simulink library "csu_afm_aerodynamics_lib"  (R2014b)
settings: Solver=ode45  StartTime=0.0  StopTime=10.0  RelTol=1e-3
values from neighbouring files (symbols this model uses):
  AeroData =     [AeroData.mat]
  afm_cg_enable = 1    [csu_afm_aerodynamics_init.m]    (also in unit_test_aero.m = 0)
  afm_forces_enable = 1    [csu_afm_aerodynamics_init.m]
  afm_gust_direction = 0.0    (= 0)    [csu_afm_aerodynamics_init.m]
  afm_gust_length = 1.0    (= 1)    [csu_afm_aerodynamics_init.m]
  afm_gust_magnitude = 0.0    (= 0)    [csu_afm_aerodynamics_init.m]
  afm_gust_number = 1    [csu_afm_aerodynamics_init.m]
  afm_gust_start = 0.0    (= 0)    [csu_afm_aerodynamics_init.m]
  afm_moments_enable = 1    [csu_afm_aerodynamics_init.m]
  afm_winds_enable = 1    [csu_afm_aerodynamics_init.m]    (also in unit_test_aero.m = 0; unit_test_winds.m)
undefined symbols (not defined in the file or in its folder): CM
libraries: simulink_need_slupdate x49, util_common_lib x17, simulink_extras x10, simulink x7, util_quat_lib x6, util_info_lib x2, util_frame_rotation_lib x2
(part 1 of 2)
settings Model: Creator=Mark Agbayani  LastModifiedBy=Mark Wells

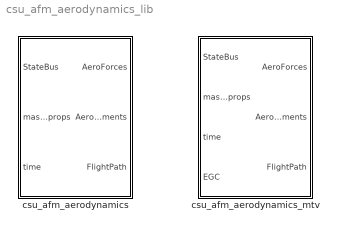
== system csu_afm_aerodynamics_lib ==
  csu_afm_aerodynamics : Subsystem
  csu_afm_aerodynamics_mtv : Subsystem

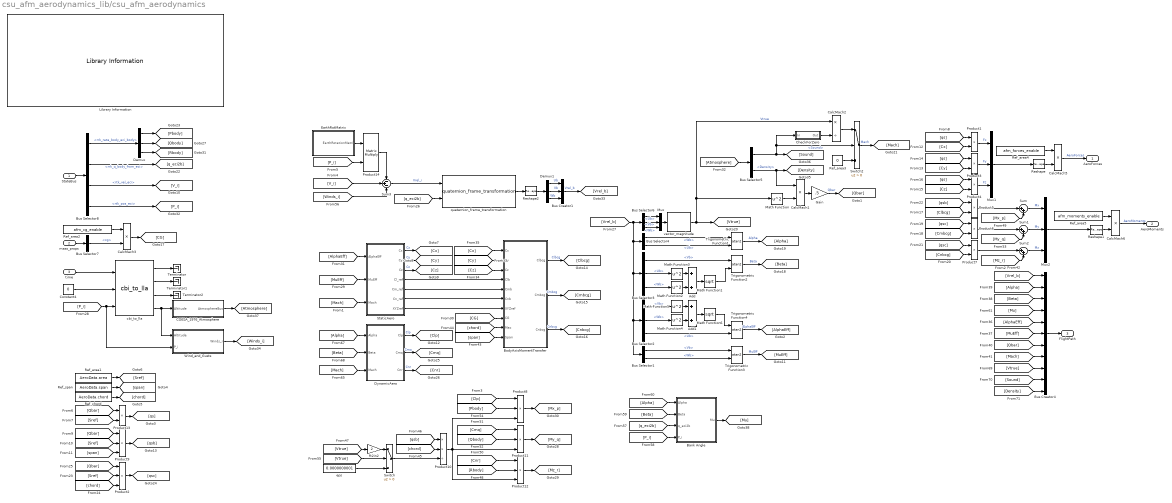
== system csu_afm_aerodynamics_lib/csu_afm_aerodynamics ==
  StateBus : Inport
  mass_props : Inport  Port=2
  time : Inport  Port=3
  Add : Sum
  Add1 : Sum
  Bank Angle : Subsystem
  BodyAxisMomentTransfer : Subsystem
  Bus Creator1 : BusCreator  Inputs=3
  Bus Creator4 : BusCreator  Inputs=11
  Bus Selector1 : BusSelector  OutputSignals=Vb,Wb
  Bus Selector2 : BusSelector  OutputSignals=Vb,Wb,Ub
  Bus Selector3 : BusSelector  OutputSignals=Vb,Ub,Wb
  Bus Selector4 : BusSelector  OutputSignals=Wb,Ub
  Bus Selector5 : BusSelector  OutputSignals=Sound,Density
  Bus Selector6 : BusSelector  OutputSignals=Ub,Vb,Wb
  Bus Selector7 : BusSelector  OutputSignals=cg
  Bus Selector8 : BusSelector  OutputSignals=rrk_rate_body_eci_body,rrk_q_body_from_eci,rtk_vel_eci,rtk_pos_eci
  COESA_1976_Atmosphere : Subsystem  mask(COESA 1976 U.S. Standard Atmosphere){}
      mask help:
      | Committee on Extension to the Standard Atmosphere (COESA) U.S. 1976 Atmosphere Model
      |
      | Computes the atmospheric values of a given geometric  altitude based on the 1976
      | U.S. Standard Atmosphere Model.  This model is valid between -5 km and 1000 km
      | (-16,404 ft and 3,280,840 ft).  Use of this block requires the associated .mat file
      | 'COESA_1976.mat'.
      |
      | Inputs:
      |        Altitude	  [m]   Geometric Altitude
      |
      | Outputs:   AtmosphereBus
      |
      |        SIGNAL NAME          UNITS       DESCRIPTION
      |        GeometricAlt         [m]         Geometric Altitude
      |        GeopotentialAlt      [m]         Geopotential Altitude
      |        Temp_Kinetic         [deg K]     Kinetic Temperature
      |        Temp_Molecular       [deg K]     Molecular Temperature
      |        Pressure             [Pa]        Atmospheric Pressure
      |        PPo                  [unitless]  Pressure / Pressure0
      |        Density              [kg/m^3]    Atmospheric Density
      |        RhoRho0              [unitless]  Rho / Rho0
      |        Sound                [m/s]       Speed of sound, Cs
      |        DynamicViscosity     [N-s/m^2]   Dynamic Viscosity, mu
      |        KinematicViscosity   [m^2/s]     Kinematic Viscosity, v
      |        kt                   [W/m-K]     Thermal Conductivity
      |        MeanFreePath         [m]          Mean Free Path
      mask init:
      | load COESA_1976.mat
      | 
      | %% Internal Variables
      | r0    = 6.356766e6;  % [m]       Radius of Earth
      | P0    = 1.013250e5;  % [N/m^2]   Standard Pressure at sea level
      | rho0  = 1.2250;      % [kg/m^3]  Standard Density at sea level
  CalcMach{1,3,5..6} (4 alike) : Product  SaturateOnIntegerOverflow=on  OutDataTypeStr=Inherit: Same as first input
  CalcMach2 : Product  Inputs=*/  SaturateOnIntegerOverflow=on  OutDataTypeStr=Inherit: Same as first input
  CheckForZero : Subsystem
  Constant4 : Constant  Value=0
  Demux : Demux  Outputs=3
  Demux1 : Demux  Outputs=3
  DynamicAero : Subsystem
  EarthRotMatrix : Subsystem
  Gain : Gain  Gain=.5
  Library Information : util_info_lib/Library Information  owner='NONE'
  Math Function{,2..5} (5 alike) : Math  Operator=square  SaturateOnIntegerOverflow=on
  Math Function1 : Math  Operator=sqrt  SaturateOnIntegerOverflow=on
  Math Function6 : Math  Operator=sqrt  SaturateOnIntegerOverflow=on
  Mux : Mux  Inputs=3
  Mux1 : Mux  Inputs=3
  Mux2 : Mux  Inputs=3
  Product{1,3..7,13} (7 alike) : Product  SaturateOnIntegerOverflow=on  OutDataTypeStr=Inherit: Same as first input
  Product10 : Product  Inputs=**/  SaturateOnIntegerOverflow=on  OutDataTypeStr=Inherit: Same as first input
  Product{2,8..9,11..12} (5 alike) : Product  Inputs=3  SaturateOnIntegerOverflow=on  OutDataTypeStr=Inherit: Same as first input
  Product14 : Product  Multiplication=Matrix(*)  SaturateOnIntegerOverflow=on  OutDataTypeStr=Inherit: Same as first input
  Ref_area1 : Constant  Value=AeroData.area
  Ref_area2 : Constant  Value=afm_cg_enable
  Ref_area3 : Constant  Value=0
  Ref_area4 : Constant  Value=afm_forces_enable
  Ref_area5 : Constant  Value=afm_moments_enable
  Ref_chord : Constant  Value=AeroData.chord
  Ref_span : Constant  Value=AeroData.span
  Reshape : Reshape
  Reshape1 : Reshape
  Reshape2 : Reshape
  StaticAero : Subsystem
  Sum : Sum  Inputs=|++  SaturateOnIntegerOverflow=on
  Sum1 : Sum  Inputs=|++  SaturateOnIntegerOverflow=on
  Sum2 : Sum  Inputs=|++  SaturateOnIntegerOverflow=on
  Sum3 : Sum  Inputs=-+-
  Switch : Switch  Criteria=u2 > Threshold  SaturateOnIntegerOverflow=on
  Switch2 : Switch  Criteria=u2 > Threshold  SaturateOnIntegerOverflow=on
  Terminator : Terminator
  Terminator1 : Terminator
  Terminator2 : Terminator
  Trigonometric Function{1..4} (4 alike) : Trigonometry  Operator=atan2
  Wind_and_Gusts : Subsystem
  cbi_to_lla : util_frame_rotation_lib/cbi_to_lla  a=6378137.0  b=6356752.314245179  omega=7.2921151467e-5
  eps : Constant  Value=0.0000000001
  ft2in2 : Gain  Gain=2  SaturateOnIntegerOverflow=on  OutDataTypeStr=Inherit: Same as input  ParamDataTypeStr=Inherit: Same as input
  quaternion_frame_transformation : util_quat_lib/quaternion_frame_transformation  SystemSampleTime=-1
  vector_magnitude : util_common_lib/vector_magnitude  SystemSampleTime=-1
  AeroForces : Outport
  AeroMoments : Outport  Port=2
  FlightPath : Outport  Port=3
  wires:
  Bus Selector7/1 -> CalcMach3/2  "<cg>"
  [Mu] -> Bus Creator4/4
  Bank Angle/1(Mu) -> [Mu]
  [Alpha] -> Bank Angle/1(Alpha)
  [Beta] -> Bank Angle/2(Beta)
  [q_eci2b] -> Bank Angle/3(q_eci2b)
  [P_i] -> Bank Angle/4(P_i)
  Switch2/1 -> [Mach]  "Mach"
  Ref_area3/1 -> Switch2/3
  CalcMach2/1 -> Switch2/1
  CheckForZero/1(Out) -> CalcMach2/2
  Reshape1/1 -> CalcMach6/2
  Ref_area5/1 -> CalcMach6/1
  Reshape/1 -> CalcMach5/2
  Ref_area4/1 -> CalcMach5/1
  Bus Selector5/1 -> [Sound], CheckForZero/1(In), Switch2/2  "<Sound>"
  Bus Selector5/2 -> CalcMach1/1, [Density]  "<Density>"
  quaternion_frame_transformation/1 -> Reshape2/1
  [Density] -> Bus Creator4/11
  [Sound] -> Bus Creator4/10
  [Vtrue] -> Bus Creator4/9
  [Mach] -> Bus Creator4/8
  [Qbar] -> Bus Creator4/7
  [MuEff] -> Bus Creator4/6
  [AlphaEff] -> Bus Creator4/5
  [Beta] -> Bus Creator4/3
  [Alpha] -> Bus Creator4/2
  [Vrel_b] -> Bus Creator4/1
  Bus Creator4/1 -> FlightPath/1
  CalcMach6/1 -> AeroMoments/1  "AeroMoments"
  CalcMach5/1 -> AeroForces/1  "AeroForces"
  [Alpha] -> DynamicAero/1(Alpha)
  [Beta] -> DynamicAero/2(Beta)
  [Mach] -> DynamicAero/3(Mach)
  Product7/1 -> Sum2/1
  DynamicAero/1(Clp) -> [Clp]  "Clp"
  [Qbar] -> Product13/1
  [Sref] -> Product13/2
  Product13/1 -> [qs]
  [Qbar] -> Product9/1
  [Sref] -> Product9/2
  [span] -> Product9/3
  Product9/1 -> [qsb]
  [qs] -> Product1/1
  [Cx] -> Product1/2
  [qs] -> Product3/1
  [Cy] -> Product3/2
  [qs] -> Product4/1
  [Cz] -> Product4/2
  Ref_area1/1 -> [Sref]
  Ref_span/1 -> [span]
  Ref_chord/1 -> [chord]
  StaticAero/1(Cx) -> [Cx]  "Cx"
  StaticAero/2(Cy) -> [Cy]  "Cy"
  StaticAero/3(Cz) -> [Cz]  "Cz"
  [Cx] -> BodyAxisMomentTransfer/1(Cx)
  [Cy] -> BodyAxisMomentTransfer/2(Cy)
  [Cz] -> BodyAxisMomentTransfer/3(Cz)
  [qsb] -> Product5/1
  [Clbcg] -> Product5/2
  [qsc] -> Product6/1
  [Cmbcg] -> Product6/2
  [qsc] -> Product7/1
  [Cnbcg] -> Product7/2
  [Qbar] -> Product2/1
  [Sref] -> Product2/2
  [chord] -> Product2/3
  Product2/1 -> [qsc]
  BodyAxisMomentTransfer/1(Clbcg) -> [Clbcg]  "Clbcg"
  BodyAxisMomentTransfer/2(Cmbcg) -> [Cmbcg]  "Cmbcg"
  BodyAxisMomentTransfer/3(Cnbcg) -> [Cnbcg]  "Cnbcg"
  [chord] -> BodyAxisMomentTransfer/9(Mac)
  [span] -> BodyAxisMomentTransfer/10(Span)
  DynamicAero/2(Cmq) -> [Cmq]  "Cmq"
  DynamicAero/3(Cnr) -> [Cnr]  "Cnr"
  Product5/1 -> Sum/1
  Product6/1 -> Sum1/1
  Sum1/1 -> Mux2/2  "My"
  Sum2/1 -> Mux2/3  "Mz"
  Product1/1 -> Mux1/1  "Fx"
  Product3/1 -> Mux1/2  "Fy"
  Product4/1 -> Mux1/3  "Fz"
  Mux1/1 -> Reshape/1
  Sum/1 -> Mux2/1  "Mx"
  [Mx_p] -> Sum/2
  [My_q] -> Sum1/2
  [Mz_r] -> Sum2/2
  [Pbody] -> Product8/2
  [Clp] -> Product8/1
  [Cmq] -> Product11/1
  [Qbody] -> Product11/2
  Product11/1 -> [My_q]
  Product12/1 -> [Mz_r]
  Product10/1 -> Product8/3, Product12/3, Product11/3
  Mux2/1 -> Reshape1/1
  StaticAero/7(XYZref) -> BodyAxisMomentTransfer/7(XYZref)
  StaticAero/4(Cl_ref) -> BodyAxisMomentTransfer/4(Clb)
  StaticAero/5(Cm_ref) -> BodyAxisMomentTransfer/5(Cmb)
  StaticAero/6(Cn_ref) -> BodyAxisMomentTransfer/6(Cnb)
  [CG] -> BodyAxisMomentTransfer/8(CG)
  vector_magnitude/1 -> [Vtrue], Math Function/1, CalcMach2/1  "Vtrue"
  CalcMach1/1 -> Gain/1
  Gain/1 -> [Qbar]  "Qbar"
  Bus Selector3/3 -> Math Function2/1  "<Wb>"
  Bus Selector3/2 -> Math Function3/1  "<Ub>"
  Math Function3/1 -> Add/1
  Math Function2/1 -> Add/2
  Add/1 -> Math Function1/1
  Bus Selector3/1 -> Trigonometric Function2/1  "<Vb>"
  Math Function1/1 -> Trigonometric Function2/2
  Trigonometric Function2/1 -> [Beta]  "Beta"
  [Mach] -> StaticAero/3(Mach)
  [MuEff] -> StaticAero/2(MuEff)
  [AlphaEff] -> StaticAero/1(AlphaEff)
  Math Function6/1 -> Trigonometric Function4/1
  Trigonometric Function3/1 -> [MuEff]  "MuEff"
  Trigonometric Function4/1 -> [AlphaEff]  "AlphaEff"
  Bus Selector2/3 -> Trigonometric Function4/2  "<Ub>"
  Bus Selector1/1 -> Trigonometric Function3/1  "<Vb>"
  Bus Selector1/2 -> Trigonometric Function3/2  "<Wb>"
  Math Function5/1 -> Add1/1
  Math Function4/1 -> Add1/2
  Add1/1 -> Math Function6/1
  Bus Selector2/1 -> Math Function5/1  "<Vb>"
  Bus Selector2/2 -> Math Function4/1  "<Wb>"
  Bus Selector4/1 -> Trigonometric Function1/1  "<Wb>"
  Bus Selector4/2 -> Trigonometric Function1/2  "<Ub>"
  Trigonometric Function1/1 -> [Alpha]  "Alpha"
  [Atmosphere] -> Bus Selector5/1
  Math Function/1 -> CalcMach1/2
  Demux/1 -> [Pbody]
  Demux/2 -> [Qbody]
  Demux/3 -> [Rbody]
  Bus Selector8/1 -> Demux/1  "<rrk_rate_body_eci_body>"
  StateBus/1 -> Bus Selector8/1
  Reshape2/1 -> Demux1/1
  Demux1/1 -> Bus Creator1/1  "Ub"
  Demux1/2 -> Bus Creator1/2  "Vb"
  Demux1/3 -> Bus Creator1/3  "Wb"
  Bus Creator1/1 -> [Vrel_b]  "Vrel_b"
  Sum3/1 -> quaternion_frame_transformation/1  "Vrel_i"
  [V_i] -> Sum3/2
  Product14/1 -> Sum3/1
  [P_i] -> Product14/2
  [q_eci2b] -> quaternion_frame_transformation/2
  EarthRotMatrix/1(EarthRotationMatrix) -> Product14/1
  CalcMach3/1 -> [CG]
  cbi_to_lla/4 -> Wind_and_Gusts/1(Altitude), COESA_1976_Atmosphere/1(Altitude)
  cbi_to_lla/1 -> Terminator/1
  cbi_to_lla/2 -> Terminator1/1
  cbi_to_lla/3 -> Terminator2/1
  COESA_1976_Atmosphere/1(AtmosphereBus) -> [Atmosphere]
  Constant4/1 -> cbi_to_lla/2
  time/1 -> cbi_to_lla/1
  [Cnr] -> Product12/1
  [Rbody] -> Product12/2
  Product8/1 -> [Mx_p]
  Bus Selector8/4 -> [P_i]  "<rtk_pos_eci>"
  Bus Selector8/2 -> [q_eci2b]  "<rrk_q_body_from_eci>"
  Bus Selector8/3 -> [V_i]  "<rtk_vel_eci>"
  Wind_and_Gusts/1(Winds_i) -> [Winds_i]
  [P_i] -> Wind_and_Gusts/2(P_i), cbi_to_lla/3
  [Winds_i] -> Sum3/3
  Ref_area2/1 -> CalcMach3/1
  mass_props/1 -> Bus Selector7/1
  eps/1 -> Switch/3
  [Vtrue] -> Switch/2
  ft2in2/1 -> Switch/1
  [Vtrue] -> ft2in2/1
  [qsb] -> Product10/1
  [chord] -> Product10/2
  Switch/1 -> Product10/3
  [Vrel_b] -> Bus Selector6/1, Bus Selector1/1, Bus Selector2/1, Bus Selector3/1, Bus Selector4/1
  Bus Selector6/1 -> Mux/1  "<Ub>"
  Bus Selector6/2 -> Mux/2  "<Vb>"
  Bus Selector6/3 -> Mux/3  "<Wb>"
  Mux/1 -> vector_magnitude/1

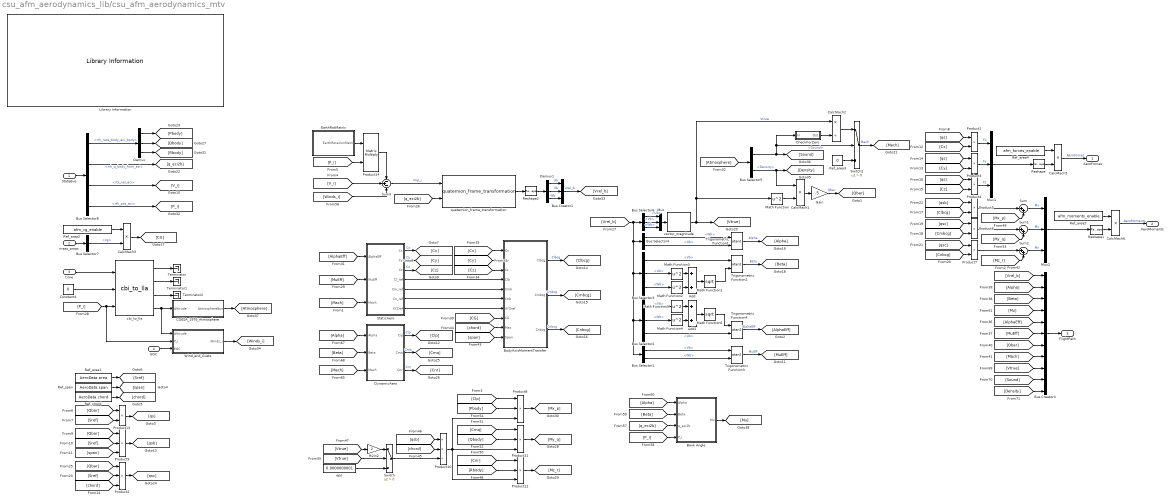
== system csu_afm_aerodynamics_lib/csu_afm_aerodynamics_mtv ==
  StateBus : Inport
  mass_props : Inport  Port=2
  time : Inport  Port=3
  EGC : Inport  Port=4
  Add : Sum
  Add1 : Sum
  Bank Angle : Subsystem
  BodyAxisMomentTransfer : Subsystem
  Bus Creator1 : BusCreator  Inputs=3
  Bus Creator4 : BusCreator  Inputs=11
  Bus Selector1 : BusSelector  OutputSignals=Vb,Wb
  Bus Selector2 : BusSelector  OutputSignals=Vb,Wb,Ub
  Bus Selector3 : BusSelector  OutputSignals=Vb,Ub,Wb
  Bus Selector4 : BusSelector  OutputSignals=Wb,Ub
  Bus Selector5 : BusSelector  OutputSignals=Sound,Density
  Bus Selector6 : BusSelector  OutputSignals=Ub,Vb,Wb
  Bus Selector7 : BusSelector  OutputSignals=cg
  Bus Selector8 : BusSelector  OutputSignals=rrk_rate_body_eci_body,rrk_q_body_from_eci,rtk_vel_eci,rtk_pos_eci
  COESA_1976_Atmosphere : Subsystem  mask(COESA 1976 U.S. Standard Atmosphere){}
      mask help:
      | Committee on Extension to the Standard Atmosphere (COESA) U.S. 1976 Atmosphere Model
      |
      | Computes the atmospheric values of a given geometric  altitude based on the 1976
      | U.S. Standard Atmosphere Model.  This model is valid between -5 km and 1000 km
      | (-16,404 ft and 3,280,840 ft).  Use of this block requires the associated .mat file
      | 'COESA_1976.mat'.
      |
      | Inputs:
      |        Altitude	  [m]   Geometric Altitude
      |
      | Outputs:   AtmosphereBus
      |
      |        SIGNAL NAME          UNITS       DESCRIPTION
      |        GeometricAlt         [m]         Geometric Altitude
      |        GeopotentialAlt      [m]         Geopotential Altitude
      |        Temp_Kinetic         [deg K]     Kinetic Temperature
      |        Temp_Molecular       [deg K]     Molecular Temperature
      |        Pressure             [Pa]        Atmospheric Pressure
      |        PPo                  [unitless]  Pressure / Pressure0
      |        Density              [kg/m^3]    Atmospheric Density
      |        RhoRho0              [unitless]  Rho / Rho0
      |        Sound                [m/s]       Speed of sound, Cs
      |        DynamicViscosity     [N-s/m^2]   Dynamic Viscosity, mu
      |        KinematicViscosity   [m^2/s]     Kinematic Viscosity, v
      |        kt                   [W/m-K]     Thermal Conductivity
      |        MeanFreePath         [m]          Mean Free Path
      mask init: same as csu_afm_aerodynamics_lib/csu_afm_aerodynamics/COESA_1976_Atmosphere
  CalcMach{1,3,5..6} (4 alike) : Product  SaturateOnIntegerOverflow=on  OutDataTypeStr=Inherit: Same as first input
  CalcMach2 : Product  Inputs=*/  SaturateOnIntegerOverflow=on  OutDataTypeStr=Inherit: Same as first input
  CheckForZero : Subsystem
  Constant4 : Constant  Value=0
  Demux : Demux  Outputs=3
  Demux1 : Demux  Outputs=3
  DynamicAero : Subsystem
  EarthRotMatrix : Subsystem
  Gain : Gain  Gain=.5
  Library Information : util_info_lib/Library Information  owner='NONE'
  Math Function{,2..5} (5 alike) : Math  Operator=square  SaturateOnIntegerOverflow=on
  Math Function1 : Math  Operator=sqrt  SaturateOnIntegerOverflow=on
  Math Function6 : Math  Operator=sqrt  SaturateOnIntegerOverflow=on
  Mux : Mux  Inputs=3
  Mux1 : Mux  Inputs=3
  Mux2 : Mux  Inputs=3
  Product{1,3..7,13} (7 alike) : Product  SaturateOnIntegerOverflow=on  OutDataTypeStr=Inherit: Same as first input
  Product10 : Product  Inputs=**/  SaturateOnIntegerOverflow=on  OutDataTypeStr=Inherit: Same as first input
  Product{2,8..9,11..12} (5 alike) : Product  Inputs=3  SaturateOnIntegerOverflow=on  OutDataTypeStr=Inherit: Same as first input
  Product14 : Product  Multiplication=Matrix(*)  SaturateOnIntegerOverflow=on  OutDataTypeStr=Inherit: Same as first input
  Ref_area1 : Constant  Value=AeroData.area
  Ref_area2 : Constant  Value=afm_cg_enable
  Ref_area3 : Constant  Value=0
  Ref_area4 : Constant  Value=afm_forces_enable
  Ref_area5 : Constant  Value=afm_moments_enable
  Ref_chord : Constant  Value=AeroData.chord
  Ref_span : Constant  Value=AeroData.span
  Reshape : Reshape
  Reshape1 : Reshape
  Reshape2 : Reshape
  StaticAero : Subsystem
  Sum : Sum  Inputs=|++  SaturateOnIntegerOverflow=on
  Sum1 : Sum  Inputs=|++  SaturateOnIntegerOverflow=on
  Sum2 : Sum  Inputs=|++  SaturateOnIntegerOverflow=on
  Sum3 : Sum  Inputs=-+-
  Switch : Switch  Criteria=u2 > Threshold  SaturateOnIntegerOverflow=on
  Switch2 : Switch  Criteria=u2 > Threshold  SaturateOnIntegerOverflow=on
  Terminator : Terminator
  Terminator1 : Terminator
  Terminator2 : Terminator
  Trigonometric Function{1..4} (4 alike) : Trigonometry  Operator=atan2
  Wind_and_Gusts : Subsystem
  cbi_to_lla : util_frame_rotation_lib/cbi_to_lla  a=6378137.0  b=6356752.314245179  omega=7.2921151467e-5
  eps : Constant  Value=0.0000000001
  ft2in2 : Gain  Gain=2  SaturateOnIntegerOverflow=on  OutDataTypeStr=Inherit: Same as input  ParamDataTypeStr=Inherit: Same as input
  quaternion_frame_transformation : util_quat_lib/quaternion_frame_transformation  SystemSampleTime=-1
  vector_magnitude : util_common_lib/vector_magnitude  SystemSampleTime=-1
  AeroForces : Outport
  AeroMoments : Outport  Port=2
  FlightPath : Outport  Port=3
  wires:
  Mux/1 -> vector_magnitude/1
  Bus Selector6/3 -> Mux/3  "<Wb>"
  Bus Selector6/2 -> Mux/2  "<Vb>"
  Bus Selector6/1 -> Mux/1  "<Ub>"
  [Vrel_b] -> Bus Selector4/1, Bus Selector3/1, Bus Selector2/1, Bus Selector1/1, Bus Selector6/1
  Switch/1 -> Product10/3
  [chord] -> Product10/2
  [qsb] -> Product10/1
  [Vtrue] -> ft2in2/1
  ft2in2/1 -> Switch/1
  [Vtrue] -> Switch/2
  eps/1 -> Switch/3
  mass_props/1 -> Bus Selector7/1
  Ref_area2/1 -> CalcMach3/1
  [Winds_i] -> Sum3/3
  [P_i] -> cbi_to_lla/3, Wind_and_Gusts/2(P_i)
  Wind_and_Gusts/1(Winds_i) -> [Winds_i]
  Bus Selector8/3 -> [V_i]  "<rtk_vel_eci>"
  Bus Selector8/2 -> [q_eci2b]  "<rrk_q_body_from_eci>"
  Bus Selector8/4 -> [P_i]  "<rtk_pos_eci>"
  Product8/1 -> [Mx_p]
  [Rbody] -> Product12/2
  [Cnr] -> Product12/1
  time/1 -> cbi_to_lla/1
  Constant4/1 -> cbi_to_lla/2
  COESA_1976_Atmosphere/1(AtmosphereBus) -> [Atmosphere]
  cbi_to_lla/3 -> Terminator2/1
  cbi_to_lla/2 -> Terminator1/1
  cbi_to_lla/1 -> Terminator/1
  cbi_to_lla/4 -> COESA_1976_Atmosphere/1(Altitude), Wind_and_Gusts/1(Altitude)
  CalcMach3/1 -> [CG]
  EarthRotMatrix/1(EarthRotationMatrix) -> Product14/1
  [q_eci2b] -> quaternion_frame_transformation/2
  [P_i] -> Product14/2
  Product14/1 -> Sum3/1
  [V_i] -> Sum3/2
  Sum3/1 -> quaternion_frame_transformation/1  "Vrel_i"
  Bus Creator1/1 -> [Vrel_b]  "Vrel_b"
  Demux1/3 -> Bus Creator1/3  "Wb"
  Demux1/2 -> Bus Creator1/2  "Vb"
  Demux1/1 -> Bus Creator1/1  "Ub"
  Reshape2/1 -> Demux1/1
  StateBus/1 -> Bus Selector8/1
  Bus Selector8/1 -> Demux/1  "<rrk_rate_body_eci_body>"
  Demux/3 -> [Rbody]
  Demux/2 -> [Qbody]
  Demux/1 -> [Pbody]
  Math Function/1 -> CalcMach1/2
  [Atmosphere] -> Bus Selector5/1
  Trigonometric Function1/1 -> [Alpha]  "Alpha"
  Bus Selector4/2 -> Trigonometric Function1/2  "<Ub>"
  Bus Selector4/1 -> Trigonometric Function1/1  "<Wb>"
  Bus Selector2/2 -> Math Function4/1  "<Wb>"
  Bus Selector2/1 -> Math Function5/1  "<Vb>"
  Add1/1 -> Math Function6/1
  Math Function4/1 -> Add1/2
  Math Function5/1 -> Add1/1
  Bus Selector1/2 -> Trigonometric Function3/2  "<Wb>"
  Bus Selector1/1 -> Trigonometric Function3/1  "<Vb>"
  Bus Selector2/3 -> Trigonometric Function4/2  "<Ub>"
  Trigonometric Function4/1 -> [AlphaEff]  "AlphaEff"
  Trigonometric Function3/1 -> [MuEff]  "MuEff"
  Math Function6/1 -> Trigonometric Function4/1
  [AlphaEff] -> StaticAero/1(AlphaEff)
  [MuEff] -> StaticAero/2(MuEff)
  [Mach] -> StaticAero/3(Mach)
  Trigonometric Function2/1 -> [Beta]  "Beta"
  Math Function1/1 -> Trigonometric Function2/2
  Bus Selector3/1 -> Trigonometric Function2/1  "<Vb>"
  Add/1 -> Math Function1/1
  Math Function2/1 -> Add/2
  Math Function3/1 -> Add/1
  Bus Selector3/2 -> Math Function3/1  "<Ub>"
  Bus Selector3/3 -> Math Function2/1  "<Wb>"
  Gain/1 -> [Qbar]  "Qbar"
  CalcMach1/1 -> Gain/1
  vector_magnitude/1 -> CalcMach2/1, Math Function/1, [Vtrue]  "Vtrue"
  [CG] -> BodyAxisMomentTransfer/8(CG)
  StaticAero/6(Cn_ref) -> BodyAxisMomentTransfer/6(Cnb)
  StaticAero/5(Cm_ref) -> BodyAxisMomentTransfer/5(Cmb)
  StaticAero/4(Cl_ref) -> BodyAxisMomentTransfer/4(Clb)
  StaticAero/7(XYZref) -> BodyAxisMomentTransfer/7(XYZref)
  Mux2/1 -> Reshape1/1
  Product10/1 -> Product11/3, Product12/3, Product8/3
  Product12/1 -> [Mz_r]
  Product11/1 -> [My_q]
  [Qbody] -> Product11/2
  [Cmq] -> Product11/1
  [Clp] -> Product8/1
  [Pbody] -> Product8/2
  [Mz_r] -> Sum2/2
  [My_q] -> Sum1/2
  [Mx_p] -> Sum/2
  Sum/1 -> Mux2/1  "Mx"
  Mux1/1 -> Reshape/1
  Product4/1 -> Mux1/3  "Fz"
  Product3/1 -> Mux1/2  "Fy"
  Product1/1 -> Mux1/1  "Fx"
  Sum2/1 -> Mux2/3  "Mz"
  Sum1/1 -> Mux2/2  "My"
  Product6/1 -> Sum1/1
  Product5/1 -> Sum/1
  DynamicAero/3(Cnr) -> [Cnr]  "Cnr"
  DynamicAero/2(Cmq) -> [Cmq]  "Cmq"
  [span] -> BodyAxisMomentTransfer/10(Span)
  [chord] -> BodyAxisMomentTransfer/9(Mac)
  BodyAxisMomentTransfer/3(Cnbcg) -> [Cnbcg]  "Cnbcg"
  BodyAxisMomentTransfer/2(Cmbcg) -> [Cmbcg]  "Cmbcg"
  BodyAxisMomentTransfer/1(Clbcg) -> [Clbcg]  "Clbcg"
  Product2/1 -> [qsc]
  [chord] -> Product2/3
  [Sref] -> Product2/2
  [Qbar] -> Product2/1
  [Cnbcg] -> Product7/2
  [qsc] -> Product7/1
  [Cmbcg] -> Product6/2
  [qsc] -> Product6/1
  [Clbcg] -> Product5/2
  [qsb] -> Product5/1
  [Cz] -> BodyAxisMomentTransfer/3(Cz)
  [Cy] -> BodyAxisMomentTransfer/2(Cy)
  [Cx] -> BodyAxisMomentTransfer/1(Cx)
  StaticAero/3(Cz) -> [Cz]  "Cz"
  StaticAero/2(Cy) -> [Cy]  "Cy"
  StaticAero/1(Cx) -> [Cx]  "Cx"
  Ref_chord/1 -> [chord]
  Ref_span/1 -> [span]
  Ref_area1/1 -> [Sref]
  [Cz] -> Product4/2
  [qs] -> Product4/1
  [Cy] -> Product3/2
  [qs] -> Product3/1
  [Cx] -> Product1/2
  [qs] -> Product1/1
  Product9/1 -> [qsb]
  [span] -> Product9/3
  [Sref] -> Product9/2
  [Qbar] -> Product9/1
  Product13/1 -> [qs]
  [Sref] -> Product13/2
  [Qbar] -> Product13/1
  DynamicAero/1(Clp) -> [Clp]  "Clp"
  Product7/1 -> Sum2/1
  [Mach] -> DynamicAero/3(Mach)
  [Beta] -> DynamicAero/2(Beta)
  [Alpha] -> DynamicAero/1(Alpha)
  CalcMach5/1 -> AeroForces/1  "AeroForces"
  CalcMach6/1 -> AeroMoments/1  "AeroMoments"
  Bus Creator4/1 -> FlightPath/1
  [Vrel_b] -> Bus Creator4/1
  [Alpha] -> Bus Creator4/2
  [Beta] -> Bus Creator4/3
  [AlphaEff] -> Bus Creator4/5
  [MuEff] -> Bus Creator4/6
  [Qbar] -> Bus Creator4/7
  [Mach] -> Bus Creator4/8
  [Vtrue] -> Bus Creator4/9
  [Sound] -> Bus Creator4/10
  [Density] -> Bus Creator4/11
  quaternion_frame_transformation/1 -> Reshape2/1
  Bus Selector5/2 -> [Density], CalcMach1/1  "<Density>"
  Bus Selector5/1 -> Switch2/2, CheckForZero/1(In), [Sound]  "<Sound>"
  Ref_area4/1 -> CalcMach5/1
  Reshape/1 -> CalcMach5/2
  Ref_area5/1 -> CalcMach6/1
  Reshape1/1 -> CalcMach6/2
  CheckForZero/1(Out) -> CalcMach2/2
  CalcMach2/1 -> Switch2/1
  Ref_area3/1 -> Switch2/3
  Switch2/1 -> [Mach]  "Mach"
  [P_i] -> Bank Angle/4(P_i)
  [q_eci2b] -> Bank Angle/3(q_eci2b)
  [Beta] -> Bank Angle/2(Beta)
  [Alpha] -> Bank Angle/1(Alpha)
  Bank Angle/1(Mu) -> [Mu]
  [Mu] -> Bus Creator4/4
  Bus Selector7/1 -> CalcMach3/2  "<cg>"
  EGC/1 -> Wind_and_Gusts/3(EGC)

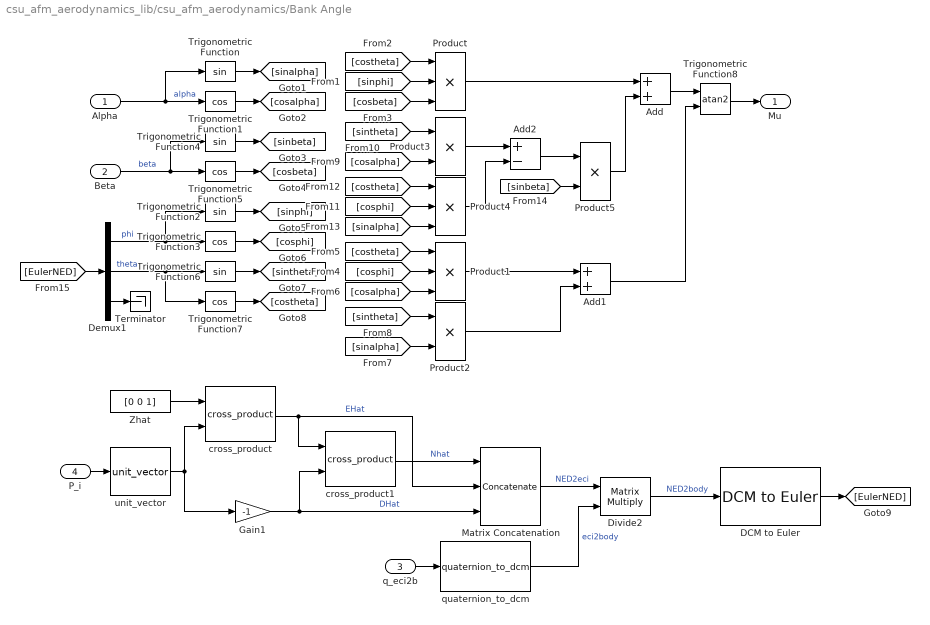
== system csu_afm_aerodynamics_lib/csu_afm_aerodynamics/Bank Angle ==
  Alpha : Inport
  Beta : Inport  Port=2
  q_eci2b : Inport  Port=3
  P_i : Inport  Port=4  PortDimensions=3
  Add : Sum
  Add1 : Sum
  Add2 : Sum  Inputs=+-
  DCM to Euler : util_quat_lib/DCM to Euler  SystemSampleTime=-1
  Demux1 : Demux  Outputs=3
  Divide2 : Product  Inputs=**  Multiplication=Matrix(*)
  Gain1 : Gain  Gain=-1
  Matrix Concatenation : Concatenate  NumInputs=3  Mode=Multidimensional array  ConcatenateDimension=2
  Product : Product  Inputs=3  RndMeth=Zero
  Product1 : Product  Inputs=3  RndMeth=Zero
  Product2 : Product  RndMeth=Zero
  Product3 : Product  RndMeth=Zero
  Product4 : Product  Inputs=3  RndMeth=Zero
  Product5 : Product  RndMeth=Zero
  Terminator : Terminator
  Trigonometric Function{,2,4,6} (4 alike) : Trigonometry
  Trigonometric Function{1,3,5,7} (4 alike) : Trigonometry  Operator=cos
  Trigonometric Function8 : Trigonometry  Operator=atan2
  Zhat : Constant  Value=[0 0 1]
  cross_product : util_common_lib/cross_product  SystemSampleTime=-1
  cross_product1 : util_common_lib/cross_product  SystemSampleTime=-1
  quaternion_to_dcm : util_quat_lib/quaternion_to_dcm  SystemSampleTime=-1
  unit_vector : util_common_lib/unit_vector  SystemSampleTime=-1
  Mu : Outport
  wires:
  [EulerNED] -> Demux1/1
  DCM to Euler/1 -> [EulerNED]
  quaternion_to_dcm/1 -> Divide2/2  "eci2body"
  q_eci2b/1 -> quaternion_to_dcm/1
  Gain1/1 -> Matrix Concatenation/3, cross_product1/2  "DHat"
  cross_product/1 -> Matrix Concatenation/2, cross_product1/1  "EHat"
  cross_product1/1 -> Matrix Concatenation/1  "Nhat"
  Matrix Concatenation/1 -> Divide2/1  "NED2eci"
  unit_vector/1 -> Gain1/1, cross_product/2
  Zhat/1 -> cross_product/1
  P_i/1 -> unit_vector/1
  Divide2/1 -> DCM to Euler/1  "NED2body"
  Demux1/1 -> Trigonometric Function3/1, Trigonometric Function2/1  "phi"
  Demux1/3 -> Terminator/1
  Demux1/2 -> Trigonometric Function6/1, Trigonometric Function7/1  "theta"
  Alpha/1 -> Trigonometric Function/1, Trigonometric Function1/1  "alpha"
  Beta/1 -> Trigonometric Function4/1, Trigonometric Function5/1  "beta"
  Trigonometric Function/1 -> [sinalpha]
  Trigonometric Function1/1 -> [cosalpha]
  Trigonometric Function4/1 -> [sinbeta]
  Trigonometric Function5/1 -> [cosbeta]
  Trigonometric Function2/1 -> [sinphi]
  Trigonometric Function3/1 -> [cosphi]
  Trigonometric Function6/1 -> [sintheta]
  Trigonometric Function7/1 -> [costheta]
  [costheta] -> Product/1
  [sinphi] -> Product/2
  [cosbeta] -> Product/3
  [costheta] -> Product1/1
  [cosphi] -> Product1/2
  [cosalpha] -> Product1/3
  Product1/1 -> Add1/1
  [sintheta] -> Product2/1
  [sinalpha] -> Product2/2
  Product2/1 -> Add1/2
  Product/1 -> Add/1
  [sintheta] -> Product3/1
  [cosalpha] -> Product3/2
  Product3/1 -> Add2/1
  [costheta] -> Product4/1
  [cosphi] -> Product4/2
  [sinalpha] -> Product4/3
  Product4/1 -> Add2/2
  Add2/1 -> Product5/1
  [sinbeta] -> Product5/2
  Product5/1 -> Add/2
  Add/1 -> Trigonometric Function8/1
  Add1/1 -> Trigonometric Function8/2
  Trigonometric Function8/1 -> Mu/1

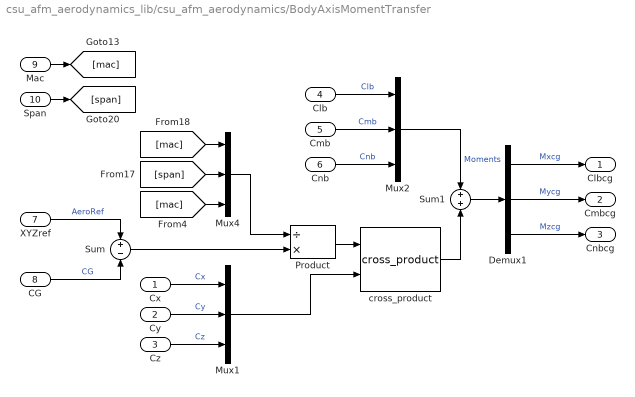
== system csu_afm_aerodynamics_lib/csu_afm_aerodynamics/BodyAxisMomentTransfer ==
  Cx : Inport
  Cy : Inport  Port=2
  Cz : Inport  Port=3
  Clb : Inport  Port=4
  Cmb : Inport  Port=5
  Cnb : Inport  Port=6
  XYZref : Inport  Port=7
  CG : Inport  Port=8
  Mac : Inport  Port=9
  Span : Inport  Port=10
  Demux1 : Demux  Outputs=3
  Mux1 : Mux  Inputs=3
  Mux2 : Mux  Inputs=3
  Mux4 : Mux  Inputs=3
  Product : Product  Inputs=/*  SaturateOnIntegerOverflow=on  OutDataTypeStr=Inherit: Same as first input
  Sum : Sum  Inputs=+-  SaturateOnIntegerOverflow=on
  Sum1 : Sum  SaturateOnIntegerOverflow=on
  cross_product : util_common_lib/cross_product  SystemSampleTime=-1
  Clbcg : Outport
  Cmbcg : Outport  Port=2
  Cnbcg : Outport  Port=3
  wires:
  Cnb/1 -> Mux2/3  "Cnb"
  Cmb/1 -> Mux2/2  "Cmb"
  Clb/1 -> Mux2/1  "Clb"
  Cz/1 -> Mux1/3  "Cz"
  Cy/1 -> Mux1/2  "Cy"
  Cx/1 -> Mux1/1  "Cx"
  Sum1/1 -> Demux1/1
  cross_product/1 -> Sum1/2
  Mux2/1 -> Sum1/1  "Moments"
  Demux1/3 -> Cnbcg/1  "Mzcg"
  Demux1/2 -> Cmbcg/1  "Mycg"
  Demux1/1 -> Clbcg/1  "Mxcg"
  Sum/1 -> Product/2
  CG/1 -> Sum/2  "CG"
  XYZref/1 -> Sum/1  "AeroRef"
  Span/1 -> [span]
  Mac/1 -> [mac]
  [mac] -> Mux4/3
  [span] -> Mux4/2
  [mac] -> Mux4/1
  Mux4/1 -> Product/1
  Mux1/1 -> cross_product/2
  Product/1 -> cross_product/1

== system csu_afm_aerodynamics_lib/csu_afm_aerodynamics/COESA_1976_Atmosphere ==
  Altitude : Inport
  Alt_PreLookup : simulink_need_slupdate/PreLookup Index Search  bpData=COESA_1976.arrZ  searchMode=Binary Search  cacheBpFlag=off  outputFlag=off  IndexDataType=uint32  extrapMode=Clip to Range  rangeErrorMode=None
  Bus Creator : BusCreator  Inputs=13
  Constant1 : Constant  Value=P0
  Constant2 : Constant  Value=rho0
  Divide : Product  Inputs=*/
  Divide1 : Product  Inputs=*/
  DocBlock : simulink/Model-Wide Utilities/DocBlock  DocumentType=Text
      content=|
      | U.S. Standard Atmosphere, 1976 (COESA 1976)
      |
      | DESCRIPTION
      |    The 1976 U.S. Standard Atmosphere (COESA 1976) is an idealized,
      | steady-state representation of the earth's atmosphere from the surface
      | to 1000 km, { -5 km to 1000 km / -16,404 feet to 3,280,840 feet } as it
      | is assumed to exist in a period of moderate solar activity.
      |
      |   For the lower altitude region (-5 km to 86 km / -16404 ft to 282,152 ft),
      | simple equations can be utilized to compute the desired output values.
      | Here the gases are considered homogeneous.
      |
      |    For the upper atmospheric regions (86 km to 1000 km / 282,152 ft to
      | 3,280,840 ft), these gases undergo dissociation and diffusion.  Since the
      | gases are no longer homogeneous, more sophisticated equations are utilized
      | to correctly model values like the dominant gases' (N2, O, O2, Ar, He, H)
      | number densities.  Since integrations are used in these equations,
      | temperature and pressure computations based on these densities carry large
      | processing times.  To avoid such delays, temperature (both kinetic and
      | molecular), pressure, and air density tables have been generated at 10 m
      | (3313.6 feet) intervals using the DOS executable in Reference 2.
      |
      | NEEDED REFERENCE FILE
      |  Filename: COESA_1976.mat (Generated with 'Build_COESA_1976.m')
      |  Description: Matlab Structure Based on Data Generated by Ref 2.
      |  Form:
      |    REF_Coesa1976       {structure}             COESA 1976
      |        .AllUnits       [1x1 struct]            Units by Parameters
      |        .Description    [1x1 struct]            Description of each .arrXX
      |        .arrZ           [100501x1]  [m]         Geometric Altitude
      |        .arrT_K         [100501x1]  [deg K]     Kinetic Temperature
      |        .arrTm_K        [100501x1]  [deg K]     Molecular Temperature
      |        .arrPress       [100501x1]  [Pa]        Atmospheric Pressure
      |        .arrDensity     [100501x1]  [kg/m^3]    Atmospheric Density
      |        .arrSound       [100501x1]  [m/s]       Speed of Sound
      |        .arrmu          [100501x1]  [N-s/m^2]   Dynamic Viscosity
      |        .arreta         [100501x1]  [m^2/s]     Kinematic Viscosity
      |        .arrkt          [100501x1]  [W/(m-K)]   Coef of Thermal Conductivity
      |
      | SOURCES
      |   Reference 1:
      |    COESA (Committee on Extension to the Standard Atmosphere), U.S.
      |    Standard Atmosphere 1976, U.S. Government Printing Office,
      |    Washington, DC, October 1976.
      |
      |   Reference 2:
      |    "U.S. Standard Atmopsphere 1976"
      |    Online References found through NASA Goddard Space Flight Center
      |
      |    Main Description:
      |      http://nssdc.gsfc.nasa.gov/space/model/atmos/us_standard.html
      |    Turbo Pascal Source Code
      |      http://www.sworld.com.au/steven/space/atmosphere/
      |      Note: This website contains corrections to Reference 1
  Geopotential_Height_m : Subsystem
  Table_Density : simulink_need_slupdate/Interpolation (n-D) using PreLookup  numDimsPopupSelect=1  explicitNumDims=2  table=COESA_1976.arrDensity  interpMethod=Linear  extrapMethod=None - Clip  rangeErrorMode=None  NumSelectionDims=0
  Table_DynamicViscosity : simulink_need_slupdate/Interpolation (n-D) using PreLookup  numDimsPopupSelect=1  explicitNumDims=2  table=COESA_1976.arrmu  interpMethod=Linear  extrapMethod=None - Clip  rangeErrorMode=None  NumSelectionDims=0
  Table_KinematicViscosity : simulink_need_slupdate/Interpolation (n-D) using PreLookup  numDimsPopupSelect=1  explicitNumDims=2  table=COESA_1976.arreta  interpMethod=Linear  extrapMethod=None - Clip  rangeErrorMode=None  NumSelectionDims=0
  Table_Kinetic_Temp : simulink_need_slupdate/Interpolation (n-D) using PreLookup  numDimsPopupSelect=1  explicitNumDims=2  table=COESA_1976.arrT_K  interpMethod=Linear  extrapMethod=None - Clip  rangeErrorMode=None  NumSelectionDims=0
  Table_MeanFreePath : simulink_need_slupdate/Interpolation (n-D) using PreLookup  numDimsPopupSelect=1  explicitNumDims=2  table=COESA_1976.arrL  interpMethod=Linear  extrapMethod=None - Clip  rangeErrorMode=None  NumSelectionDims=0
  Table_Molecular_Temp : simulink_need_slupdate/Interpolation (n-D) using PreLookup  numDimsPopupSelect=1  explicitNumDims=2  table=COESA_1976.arrTm_K  interpMethod=Linear  extrapMethod=None - Clip  rangeErrorMode=None  NumSelectionDims=0
  Table_Pressure : simulink_need_slupdate/Interpolation (n-D) using PreLookup  numDimsPopupSelect=1  explicitNumDims=2  table=COESA_1976.arrPress  interpMethod=Linear  extrapMethod=None - Clip  rangeErrorMode=None  NumSelectionDims=0
  Table_SpeedofSound : simulink_need_slupdate/Interpolation (n-D) using PreLookup  numDimsPopupSelect=1  explicitNumDims=2  table=COESA_1976.arrSound  interpMethod=Linear  extrapMethod=None - Clip  rangeErrorMode=None  NumSelectionDims=0
  Table_ThermalConductivity : simulink_need_slupdate/Interpolation (n-D) using PreLookup  numDimsPopupSelect=1  explicitNumDims=2  table=COESA_1976.arrkt  interpMethod=Linear  extrapMethod=None - Clip  rangeErrorMode=None  NumSelectionDims=0
  AtmosphereBus : Outport
  wires:
  Table_Kinetic_Temp/1 -> Bus Creator/3  "Temp_Kinetic"
  Table_Molecular_Temp/1 -> Bus Creator/4  "Temp_Molecular"
  Table_Pressure/1 -> Bus Creator/5, Divide/1  "Pressure"
  Table_Density/1 -> Bus Creator/7, Divide1/1  "Density"
  Altitude/1 -> Bus Creator/1, Geopotential_Height_m/1(Z_m), Alt_PreLookup/1  "GeometricAlt"
  Geopotential_Height_m/1(H_m) -> Bus Creator/2  "GeopotentialAlt"
  Divide/1 -> Bus Creator/6  "PP0"
  Constant1/1 -> Divide/2
  Constant2/1 -> Divide1/2
  Divide1/1 -> Bus Creator/8  "RhoRho0"
  Table_DynamicViscosity/1 -> Bus Creator/10  "DynamicViscosity"
  Bus Creator/1 -> AtmosphereBus/1
  Table_MeanFreePath/1 -> Bus Creator/13  "MeanFreePath"
  Table_SpeedofSound/1 -> Bus Creator/9  "Sound"
  Table_KinematicViscosity/1 -> Bus Creator/11  "KinematicViscosity"
  Table_ThermalConductivity/1 -> Bus Creator/12  "kt"
  Alt_PreLookup/1 -> Table_Kinetic_Temp/1, Table_Molecular_Temp/1, Table_Pressure/1, Table_Density/1, Table_SpeedofSound/1, Table_DynamicViscosity/1, Table_KinematicViscosity/1, Table_ThermalConductivity/1, Table_MeanFreePath/1

== system csu_afm_aerodynamics_lib/csu_afm_aerodynamics/CheckForZero ==
  In : Inport
  Constant : Constant  Value=0
  Gain : Gain  Gain=eps
  Logical Operator1 : Logic  Operator=NOT  AllPortsSameDT=off  OutDataTypeStr=float('double')
  Product : Product  RndMeth=Zero
  Relational Operator : RelationalOperator  Operator===  OutDataTypeStr=float('double')
  Sum : Sum  Inputs=|++
  Out : Outport
  wires:
  In/1 -> Product/1, Relational Operator/1
  Relational Operator/1 -> Gain/1, Logical Operator1/1
  Gain/1 -> Sum/2
  Logical Operator1/1 -> Product/2
  Product/1 -> Sum/1
  Sum/1 -> Out/1
  Constant/1 -> Relational Operator/2

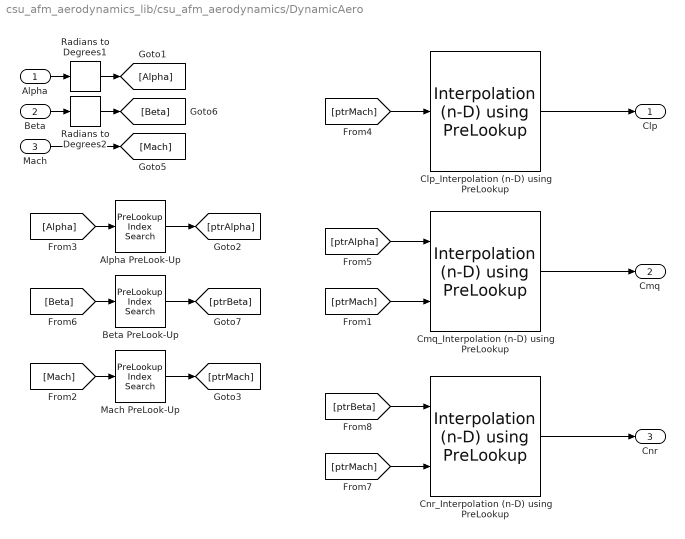
== system csu_afm_aerodynamics_lib/csu_afm_aerodynamics/DynamicAero ==
  Alpha : Inport
  Beta : Inport  Port=2
  Mach : Inport  Port=3
  Alpha PreLook-Up : simulink_need_slupdate/PreLookup Index Search  bpData=AeroData.Dynamic.Alpha  searchMode=Binary Search  cacheBpFlag=on  outputFlag=off  IndexDataType=uint32  extrapMode=Clip to Range  rangeErrorMode=None
  Beta PreLook-Up : simulink_need_slupdate/PreLookup Index Search  bpData=AeroData.Dynamic.Beta  searchMode=Binary Search  cacheBpFlag=on  outputFlag=off  IndexDataType=uint32  extrapMode=Clip to Range  rangeErrorMode=None
  Clp_Interpolation (n-D) using PreLookup : simulink_need_slupdate/Interpolation (n-D) using PreLookup  numDimsPopupSelect=1  explicitNumDims=2  table=AeroData.Dynamic.Clp  interpMethod=Linear  extrapMethod=None - Clip  rangeErrorMode=None  NumSelectionDims=0
  Cmq_Interpolation (n-D) using PreLookup : simulink_need_slupdate/Interpolation (n-D) using PreLookup  numDimsPopupSelect=2  explicitNumDims=2  table=AeroData.Dynamic.Cmq  interpMethod=Linear  extrapMethod=None - Clip  rangeErrorMode=None  NumSelectionDims=0
  Cnr_Interpolation (n-D) using PreLookup : simulink_need_slupdate/Interpolation (n-D) using PreLookup  numDimsPopupSelect=2  explicitNumDims=2  table=AeroData.Dynamic.Cnr  interpMethod=Linear  extrapMethod=None - Clip  rangeErrorMode=None  NumSelectionDims=0
  Mach PreLook-Up : simulink_need_slupdate/PreLookup Index Search  bpData=AeroData.Dynamic.Mach  searchMode=Binary Search  cacheBpFlag=on  outputFlag=off  IndexDataType=uint32  extrapMode=Clip to Range  rangeErrorMode=None
  Radians to Degrees1 : simulink_extras/Transformations/Radians to Degrees
  Radians to Degrees2 : simulink_extras/Transformations/Radians to Degrees
  Clp : Outport  PortDimensions=1  InitialOutput=CM.Aero.DynamicData.CM_only.Clp
  Cmq : Outport  Port=2  PortDimensions=1  InitialOutput=0
  Cnr : Outport  Port=3  PortDimensions=1  InitialOutput=0
  wires:
  Alpha/1 -> Radians to Degrees1/1
  Beta/1 -> Radians to Degrees2/1
  Radians to Degrees2/1 -> [Beta]
  Radians to Degrees1/1 -> [Alpha]
  Cnr_Interpolation (n-D) using PreLookup/1 -> Cnr/1
  Cmq_Interpolation (n-D) using PreLookup/1 -> Cmq/1
  [Beta] -> Beta PreLook-Up/1
  Beta PreLook-Up/1 -> [ptrBeta]
  [Mach] -> Mach PreLook-Up/1
  [Alpha] -> Alpha PreLook-Up/1
  Mach PreLook-Up/1 -> [ptrMach]
  Alpha PreLook-Up/1 -> [ptrAlpha]
  [ptrMach] -> Cnr_Interpolation (n-D) using PreLookup/2
  [ptrBeta] -> Cnr_Interpolation (n-D) using PreLookup/1
  [ptrMach] -> Cmq_Interpolation (n-D) using PreLookup/2
  [ptrAlpha] -> Cmq_Interpolation (n-D) using PreLookup/1
  Mach/1 -> [Mach]
  Clp_Interpolation (n-D) using PreLookup/1 -> Clp/1
  [ptrMach] -> Clp_Interpolation (n-D) using PreLookup/1

== system csu_afm_aerodynamics_lib/csu_afm_aerodynamics/EarthRotMatrix ==
  Constant{1..7} (7 alike) : Constant  Value=0
  EarthRate : Constant  Value=7.2921151467e-5
  Gain1 : Gain  Gain=-1  SaturateOnIntegerOverflow=on  OutDataTypeStr=Inherit: Same as input  ParamDataTypeStr=Inherit: Same as input
  Matrix Concatenation : Concatenate  NumInputs=3  Mode=Multidimensional array  ConcatenateDimension=2
  Mux : Mux  Inputs=3
  Mux1 : Mux  Inputs=3
  Mux2 : Mux  Inputs=3
  EarthRotationMatrix : Outport
  wires:
  [omegaE] -> Gain1/1
  Mux/1 -> Matrix Concatenation/1
  Mux1/1 -> Matrix Concatenation/2
  Gain1/1 -> Mux1/1
  Constant2/1 -> Mux1/3
  Constant1/1 -> Mux2/1
  Constant3/1 -> Mux2/2
  Constant7/1 -> Mux2/3
  Constant4/1 -> Mux1/2
  Constant6/1 -> Mux/3
  Constant5/1 -> Mux/1
  [omegaE] -> Mux/2
  EarthRate/1 -> [omegaE]
  Matrix Concatenation/1 -> EarthRotationMatrix/1
  Mux2/1 -> Matrix Concatenation/3

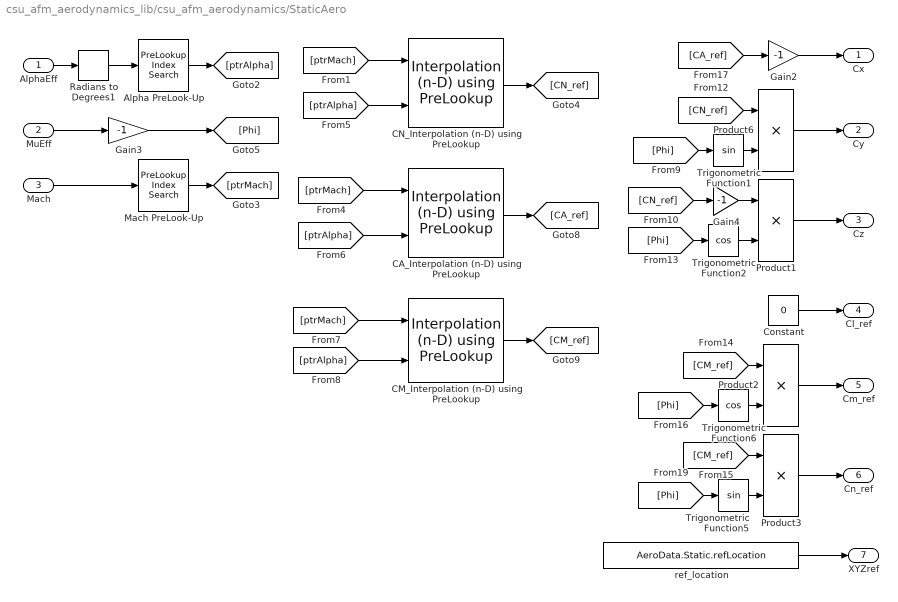
== system csu_afm_aerodynamics_lib/csu_afm_aerodynamics/StaticAero ==
  AlphaEff : Inport
  MuEff : Inport  Port=2
  Mach : Inport  Port=3
  Alpha PreLook-Up : simulink_need_slupdate/PreLookup Index Search  bpData=AeroData.Static.Alpha  searchMode=Binary Search  cacheBpFlag=on  outputFlag=off  IndexDataType=uint32  extrapMode=Clip to Range  rangeErrorMode=None
  CA_Interpolation (n-D) using PreLookup : simulink_need_slupdate/Interpolation (n-D) using PreLookup  numDimsPopupSelect=2  explicitNumDims=2  table=AeroData.Static.CA  interpMethod=Linear  extrapMethod=None - Clip  rangeErrorMode=None  NumSelectionDims=0
  CM_Interpolation (n-D) using PreLookup : simulink_need_slupdate/Interpolation (n-D) using PreLookup  numDimsPopupSelect=2  explicitNumDims=2  table=AeroData.Static.CM  interpMethod=Linear  extrapMethod=None - Clip  rangeErrorMode=None  NumSelectionDims=0
  CN_Interpolation (n-D) using PreLookup : simulink_need_slupdate/Interpolation (n-D) using PreLookup  numDimsPopupSelect=2  explicitNumDims=2  table=AeroData.Static.CN  interpMethod=Linear  extrapMethod=None - Clip  rangeErrorMode=None  NumSelectionDims=0
  Constant : Constant  Value=0
  Gain2 : Gain  Gain=-1
  Gain3 : Gain  Gain=-1
  Gain4 : Gain  Gain=-1
  Mach PreLook-Up : simulink_need_slupdate/PreLookup Index Search  bpData=AeroData.Static.Mach  searchMode=Binary Search  cacheBpFlag=on  outputFlag=off  IndexDataType=uint32  extrapMode=Clip to Range  rangeErrorMode=None
  Product{1..3,6} (4 alike) : Product  SaturateOnIntegerOverflow=on  OutDataTypeStr=Inherit: Same as first input
  Radians to Degrees1 : simulink_extras/Transformations/Radians to Degrees
  Trigonometric Function1 : Trigonometry
  Trigonometric Function2 : Trigonometry  Operator=cos
  Trigonometric Function5 : Trigonometry
  Trigonometric Function6 : Trigonometry  Operator=cos
  ref_location : Constant  Value=AeroData.Static.refLocation
  Cx : Outport
  Cy : Outport  Port=2
  Cz : Outport  Port=3
  Cl_ref : Outport  Port=4
  Cm_ref : Outport  Port=5
  Cn_ref : Outport  Port=6
  XYZref : Outport  Port=7  InitialOutput=[0 0 0]
  wires:
  Alpha PreLook-Up/1 -> [ptrAlpha]
  Mach PreLook-Up/1 -> [ptrMach]
  AlphaEff/1 -> Radians to Degrees1/1
  MuEff/1 -> Gain3/1
  CN_Interpolation (n-D) using PreLookup/1 -> [CN_ref]
  CA_Interpolation (n-D) using PreLookup/1 -> [CA_ref]
  CM_Interpolation (n-D) using PreLookup/1 -> [CM_ref]
  [CA_ref] -> Gain2/1
  [ptrMach] -> CN_Interpolation (n-D) using PreLookup/1
  [ptrAlpha] -> CN_Interpolation (n-D) using PreLookup/2
  [ptrMach] -> CA_Interpolation (n-D) using PreLookup/1
  [ptrAlpha] -> CA_Interpolation (n-D) using PreLookup/2
  [ptrMach] -> CM_Interpolation (n-D) using PreLookup/1
  [ptrAlpha] -> CM_Interpolation (n-D) using PreLookup/2
  Mach/1 -> Mach PreLook-Up/1
  Gain2/1 -> Cx/1
  Product6/1 -> Cy/1
  [Phi] -> Trigonometric Function2/1
  Trigonometric Function2/1 -> Product1/2
  Constant/1 -> Cl_ref/1
  [CN_ref] -> Product6/1
  [Phi] -> Trigonometric Function1/1
  Trigonometric Function1/1 -> Product6/2
  [CN_ref] -> Gain4/1
  Product1/1 -> Cz/1
  [Phi] -> Trigonometric Function6/1
  Trigonometric Function6/1 -> Product2/2
  [CM_ref] -> Product3/1
  [Phi] -> Trigonometric Function5/1
  Trigonometric Function5/1 -> Product3/2
  [CM_ref] -> Product2/1
  Product2/1 -> Cm_ref/1
  Product3/1 -> Cn_ref/1
  Gain3/1 -> [Phi]
  Gain4/1 -> Product1/1
  Radians to Degrees1/1 -> Alpha PreLook-Up/1
  ref_location/1 -> XYZref/1

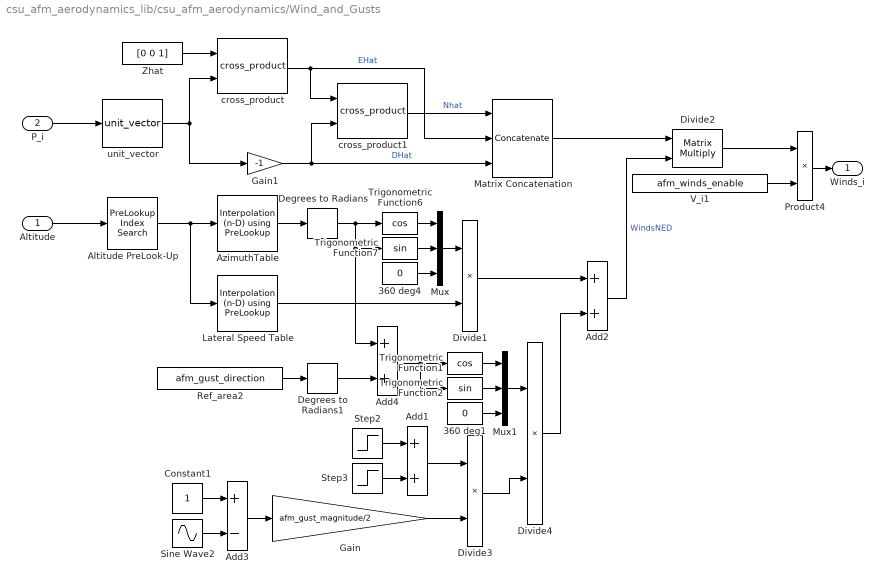
== system csu_afm_aerodynamics_lib/csu_afm_aerodynamics/Wind_and_Gusts ==
  Altitude : Inport  PortDimensions=1
  P_i : Inport  Port=2  PortDimensions=3
  360 deg1 : Constant  Value=0
  360 deg4 : Constant  Value=0
  Add1 : Sum
  Add2 : Sum
  Add3 : Sum  Inputs=+-
  Add4 : Sum
  Altitude PreLook-Up : simulink_need_slupdate/PreLookup Index Search  bpData=Winds.Altitude  searchMode=Binary Search  cacheBpFlag=on  outputFlag=off  IndexDataType=uint32  extrapMode=Clip to Range  rangeErrorMode=None
  AzimuthTable : simulink_need_slupdate/Interpolation (n-D) using PreLookup  numDimsPopupSelect=1  explicitNumDims=2  table=Winds.Azimuth  interpMethod=Linear  extrapMethod=None - Clip  rangeErrorMode=None  NumSelectionDims=0
  Constant1 : Constant
  Degrees to Radians : simulink_extras/Transformations/Degrees to Radians
  Degrees to Radians1 : simulink_extras/Transformations/Degrees to Radians
  Divide1 : Product  Inputs=**
  Divide2 : Product  Inputs=**  Multiplication=Matrix(*)
  Divide3 : Product  Inputs=**
  Divide4 : Product  Inputs=**
  Gain : Gain  Gain=afm_gust_magnitude/2
  Gain1 : Gain  Gain=-1
  Lateral Speed Table : simulink_need_slupdate/Interpolation (n-D) using PreLookup  numDimsPopupSelect=1  explicitNumDims=2  table=Winds.Speed.Lateral  interpMethod=Linear  extrapMethod=None - Clip  rangeErrorMode=None  NumSelectionDims=0
  Matrix Concatenation : Concatenate  NumInputs=3  Mode=Multidimensional array  ConcatenateDimension=2
  Mux : Mux  Inputs=3
  Mux1 : Mux  Inputs=3
  Product4 : Product  RndMeth=Zero
  Ref_area2 : Constant  Value=afm_gust_direction
  Sine Wave2 : Sin  Frequency=2*pi/afm_gust_length*afm_gust_number  Phase=pi/2-2*pi/afm_gust_length*afm_gust_number*afm_gust_start  SampleTime=.01  VectorParams1D=off
  Step2 : Step  Time=afm_gust_start  SampleTime=.01
  Step3 : Step  Time=afm_gust_start+afm_gust_length  After=-1  SampleTime=.01
  Trigonometric Function1 : Trigonometry  Operator=cos
  Trigonometric Function2 : Trigonometry
  Trigonometric Function6 : Trigonometry  Operator=cos
  Trigonometric Function7 : Trigonometry
  V_i1 : Constant  Value=afm_winds_enable  VectorParams1D=off
  Zhat : Constant  Value=[0 0 1]
  cross_product : util_common_lib/cross_product  SystemSampleTime=-1
  cross_product1 : util_common_lib/cross_product  SystemSampleTime=-1
  unit_vector : util_common_lib/unit_vector  SystemSampleTime=-1
  Winds_i : Outport  PortDimensions=3
  wires:
  Altitude PreLook-Up/1 -> Lateral Speed Table/1, AzimuthTable/1
  Altitude/1 -> Altitude PreLook-Up/1
  Trigonometric Function6/1 -> Mux/1
  Trigonometric Function7/1 -> Mux/2
  360 deg4/1 -> Mux/3
  Mux/1 -> Divide1/1
  Lateral Speed Table/1 -> Divide1/2
  Gain1/1 -> Matrix Concatenation/3, cross_product1/2  "DHat"
  cross_product/1 -> Matrix Concatenation/2, cross_product1/1  "EHat"
  cross_product1/1 -> Matrix Concatenation/1  "Nhat"
  Matrix Concatenation/1 -> Divide2/1
  Product4/1 -> Winds_i/1
  Degrees to Radians/1 -> Trigonometric Function7/1, Add4/1, Trigonometric Function6/1
  unit_vector/1 -> Gain1/1, cross_product/2
  Zhat/1 -> cross_product/1
  P_i/1 -> unit_vector/1
  AzimuthTable/1 -> Degrees to Radians/1
  V_i1/1 -> Product4/2
  Divide2/1 -> Product4/1
  Gain/1 -> Divide3/2
  Step2/1 -> Add1/1
  Step3/1 -> Add1/2
  Add1/1 -> Divide3/1
  Divide3/1 -> Divide4/2
  Add2/1 -> Divide2/2  "WindsNED"
  Constant1/1 -> Add3/1
  Add3/1 -> Gain/1
  Sine Wave2/1 -> Add3/2
  Trigonometric Function1/1 -> Mux1/1
  Trigonometric Function2/1 -> Mux1/2
  Mux1/1 -> Divide4/1
  Add4/1 -> Trigonometric Function2/1, Trigonometric Function1/1
  Ref_area2/1 -> Degrees to Radians1/1
  Degrees to Radians1/1 -> Add4/2
  360 deg1/1 -> Mux1/3
  Divide1/1 -> Add2/1
  Divide4/1 -> Add2/2

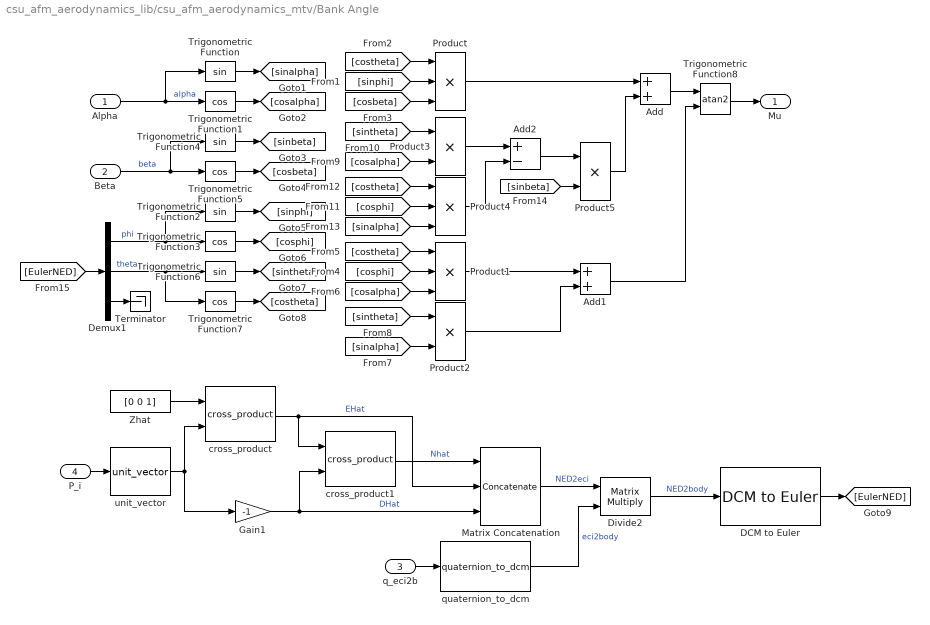
== system csu_afm_aerodynamics_lib/csu_afm_aerodynamics_mtv/Bank Angle ==
  Alpha : Inport
  Beta : Inport  Port=2
  q_eci2b : Inport  Port=3
  P_i : Inport  Port=4  PortDimensions=3
  Add : Sum
  Add1 : Sum
  Add2 : Sum  Inputs=+-
  DCM to Euler : util_quat_lib/DCM to Euler  SystemSampleTime=-1
  Demux1 : Demux  Outputs=3
  Divide2 : Product  Inputs=**  Multiplication=Matrix(*)
  Gain1 : Gain  Gain=-1
  Matrix Concatenation : Concatenate  NumInputs=3  Mode=Multidimensional array  ConcatenateDimension=2
  Product : Product  Inputs=3  RndMeth=Zero
  Product1 : Product  Inputs=3  RndMeth=Zero
  Product2 : Product  RndMeth=Zero
  Product3 : Product  RndMeth=Zero
  Product4 : Product  Inputs=3  RndMeth=Zero
  Product5 : Product  RndMeth=Zero
  Terminator : Terminator
  Trigonometric Function{,2,4,6} (4 alike) : Trigonometry
  Trigonometric Function{1,3,5,7} (4 alike) : Trigonometry  Operator=cos
  Trigonometric Function8 : Trigonometry  Operator=atan2
  Zhat : Constant  Value=[0 0 1]
  cross_product : util_common_lib/cross_product  SystemSampleTime=-1
  cross_product1 : util_common_lib/cross_product  SystemSampleTime=-1
  quaternion_to_dcm : util_quat_lib/quaternion_to_dcm  SystemSampleTime=-1
  unit_vector : util_common_lib/unit_vector  SystemSampleTime=-1
  Mu : Outport
  wires:
  Trigonometric Function8/1 -> Mu/1
  Add1/1 -> Trigonometric Function8/2
  Add/1 -> Trigonometric Function8/1
  Product5/1 -> Add/2
  [sinbeta] -> Product5/2
  Add2/1 -> Product5/1
  Product4/1 -> Add2/2
  [sinalpha] -> Product4/3
  [cosphi] -> Product4/2
  [costheta] -> Product4/1
  Product3/1 -> Add2/1
  [cosalpha] -> Product3/2
  [sintheta] -> Product3/1
  Product/1 -> Add/1
  Product2/1 -> Add1/2
  [sinalpha] -> Product2/2
  [sintheta] -> Product2/1
  Product1/1 -> Add1/1
  [cosalpha] -> Product1/3
  [cosphi] -> Product1/2
  [costheta] -> Product1/1
  [cosbeta] -> Product/3
  [sinphi] -> Product/2
  [costheta] -> Product/1
  Trigonometric Function7/1 -> [costheta]
  Trigonometric Function6/1 -> [sintheta]
  Trigonometric Function3/1 -> [cosphi]
  Trigonometric Function2/1 -> [sinphi]
  Trigonometric Function5/1 -> [cosbeta]
  Trigonometric Function4/1 -> [sinbeta]
  Trigonometric Function1/1 -> [cosalpha]
  Trigonometric Function/1 -> [sinalpha]
  Beta/1 -> Trigonometric Function5/1, Trigonometric Function4/1  "beta"
  Alpha/1 -> Trigonometric Function1/1, Trigonometric Function/1  "alpha"
  Demux1/2 -> Trigonometric Function7/1, Trigonometric Function6/1  "theta"
  Demux1/3 -> Terminator/1
  Demux1/1 -> Trigonometric Function2/1, Trigonometric Function3/1  "phi"
  Divide2/1 -> DCM to Euler/1  "NED2body"
  P_i/1 -> unit_vector/1
  Zhat/1 -> cross_product/1
  unit_vector/1 -> cross_product/2, Gain1/1
  Matrix Concatenation/1 -> Divide2/1  "NED2eci"
  cross_product1/1 -> Matrix Concatenation/1  "Nhat"
  cross_product/1 -> cross_product1/1, Matrix Concatenation/2  "EHat"
  Gain1/1 -> cross_product1/2, Matrix Concatenation/3  "DHat"
  q_eci2b/1 -> quaternion_to_dcm/1
  quaternion_to_dcm/1 -> Divide2/2  "eci2body"
  DCM to Euler/1 -> [EulerNED]
  [EulerNED] -> Demux1/1

== system csu_afm_aerodynamics_lib/csu_afm_aerodynamics_mtv/BodyAxisMomentTransfer ==
  Cx : Inport
  Cy : Inport  Port=2
  Cz : Inport  Port=3
  Clb : Inport  Port=4
  Cmb : Inport  Port=5
  Cnb : Inport  Port=6
  XYZref : Inport  Port=7
  CG : Inport  Port=8
  Mac : Inport  Port=9
  Span : Inport  Port=10
  Demux1 : Demux  Outputs=3
  Mux1 : Mux  Inputs=3
  Mux2 : Mux  Inputs=3
  Mux4 : Mux  Inputs=3
  Product : Product  Inputs=/*  SaturateOnIntegerOverflow=on  OutDataTypeStr=Inherit: Same as first input
  Sum : Sum  Inputs=+-  SaturateOnIntegerOverflow=on
  Sum1 : Sum  SaturateOnIntegerOverflow=on
  cross_product : util_common_lib/cross_product  SystemSampleTime=-1
  Clbcg : Outport
  Cmbcg : Outport  Port=2
  Cnbcg : Outport  Port=3
  wires:
  Product/1 -> cross_product/1
  Mux1/1 -> cross_product/2
  Mux4/1 -> Product/1
  [mac] -> Mux4/1
  [span] -> Mux4/2
  [mac] -> Mux4/3
  Mac/1 -> [mac]
  Span/1 -> [span]
  XYZref/1 -> Sum/1  "AeroRef"
  CG/1 -> Sum/2  "CG"
  Sum/1 -> Product/2
  Demux1/1 -> Clbcg/1  "Mxcg"
  Demux1/2 -> Cmbcg/1  "Mycg"
  Demux1/3 -> Cnbcg/1  "Mzcg"
  Mux2/1 -> Sum1/1  "Moments"
  cross_product/1 -> Sum1/2
  Sum1/1 -> Demux1/1
  Cx/1 -> Mux1/1  "Cx"
  Cy/1 -> Mux1/2  "Cy"
  Cz/1 -> Mux1/3  "Cz"
  Clb/1 -> Mux2/1  "Clb"
  Cmb/1 -> Mux2/2  "Cmb"
  Cnb/1 -> Mux2/3  "Cnb"
